simulink model "PDcontroller_simulink"  (R2018b)
settings: Solver=VariableStepAuto  StartTime=0.0  StopTime=1  RelTol=1e-3
settings Model: Creator=luonc  LastModifiedBy=luonc

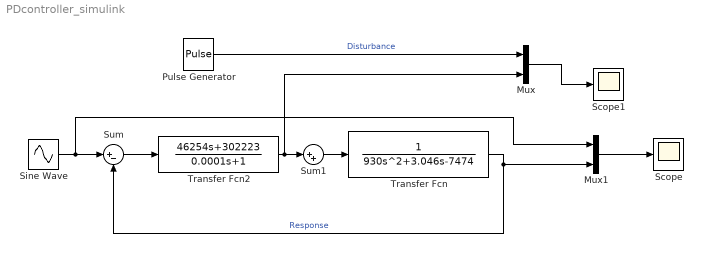
== system PDcontroller_simulink ==
  Mux : Mux  Inputs=2
  Mux1 : Mux  Inputs=2
  Pulse Generator : DiscretePulseGenerator  PulseType=Time based  Amplitude=1500  Period=1
  Scope : Scope
  Scope1 : Scope
  Sine Wave : Sin  Frequency=5*2*3.14  SampleTime=0
  Sum : Sum  Inputs=|+-
  Sum1 : Sum  Inputs=|++
  Transfer Fcn : TransferFcn  Denominator=[930 3.046 -7474]
  Transfer Fcn2 : TransferFcn  Numerator=[46254 302223]  Denominator=[0.0001 1]
  wires:
  Sum/1 -> Transfer Fcn2/1
  Transfer Fcn/1 -> Sum/2, Mux1/2  "Response"
  Sine Wave/1 -> Mux1/1, Sum/1
  Transfer Fcn2/1 -> Mux/2, Sum1/1
  Sum1/1 -> Transfer Fcn/1
  Pulse Generator/1 -> Mux/1  "Disturbance"
  Mux/1 -> Scope1/1
  Mux1/1 -> Scope/1
